simulink model "[Simulink]LA Mendoza20211984"  (R2023a)
settings: Solver=VariableStepAuto  StartTime=0.0  StopTime=10.0  RelTol=1e-3
settings Model: Creator=Marco  LastModifiedBy=Marco

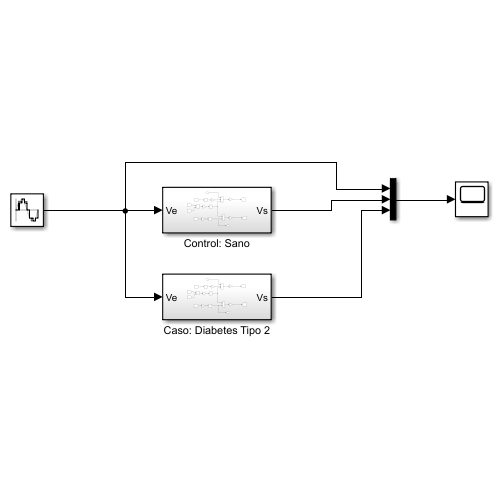
[thumbnail: Simulink's stored preview of the top-level diagram]
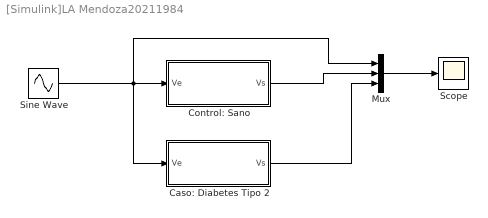
== system [Simulink]LA Mendoza20211984 ==
  Caso: Diabetes Tipo 2 : Subsystem
  Control: Sano : Subsystem
  Mux : Mux  Inputs=3
  Scope : Scope
  Sine Wave : Sin  Frequency=1.5708  SampleTime=0.001
  wires:
  Sine Wave/1 -> Caso: Diabetes Tipo 2/1(Ve), Mux/1, Control: Sano/1(Ve)
  Control: Sano/1(Vs) -> Mux/2
  Mux/1 -> Scope/1
  Caso: Diabetes Tipo 2/1(Vs) -> Mux/3

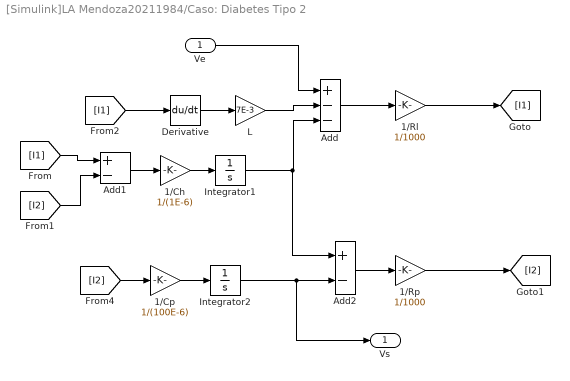
== system [Simulink]LA Mendoza20211984/Caso: Diabetes Tipo 2 ==
  Ve : Inport
  1/Ch : Gain  Gain=1/(1E-6)
  1/Cp : Gain  Gain=1/(100E-6)
  1/Rl : Gain  Gain=1/1000
  1/Rp : Gain  Gain=1/1000
  Add : Sum  Inputs=+--
  Add1 : Sum  Inputs=+-
  Add2 : Sum  Inputs=+-
  Derivative : Derivative
  Integrator1 : Integrator
  Integrator2 : Integrator
  L : Gain  Gain=7E-3
  Vs : Outport
  wires:
  Ve/1 -> Add/1
  Add1/1 -> 1/Ch/1
  [I1] -> Add1/1
  [I2] -> Add1/2
  [I1] -> Derivative/1
  Add/1 -> 1/Rl/1
  1/Rl/1 -> [I1]
  1/Ch/1 -> Integrator1/1
  Integrator1/1 -> Add2/1, Add/3
  Derivative/1 -> L/1
  L/1 -> Add/2
  [I2] -> 1/Cp/1
  1/Cp/1 -> Integrator2/1
  Integrator2/1 -> Vs/1, Add2/2
  Add2/1 -> 1/Rp/1
  1/Rp/1 -> [I2]

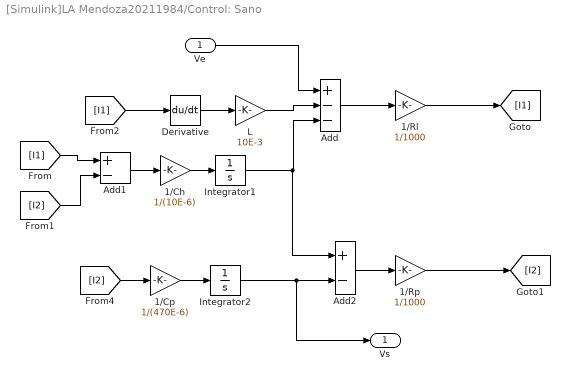
== system [Simulink]LA Mendoza20211984/Control: Sano ==
  Ve : Inport
  1/Ch : Gain  Gain=1/(10E-6)
  1/Cp : Gain  Gain=1/(470E-6)
  1/Rl : Gain  Gain=1/1000
  1/Rp : Gain  Gain=1/1000
  Add : Sum  Inputs=+--
  Add1 : Sum  Inputs=+-
  Add2 : Sum  Inputs=+-
  Derivative : Derivative
  Integrator1 : Integrator
  Integrator2 : Integrator
  L : Gain  Gain=10E-3
  Vs : Outport
  wires:
  Ve/1 -> Add/1
  Add1/1 -> 1/Ch/1
  [I1] -> Add1/1
  [I2] -> Add1/2
  [I1] -> Derivative/1
  Add/1 -> 1/Rl/1
  1/Rl/1 -> [I1]
  1/Ch/1 -> Integrator1/1
  Integrator1/1 -> Add2/1, Add/3
  Derivative/1 -> L/1
  L/1 -> Add/2
  [I2] -> 1/Cp/1
  1/Cp/1 -> Integrator2/1
  Integrator2/1 -> Vs/1, Add2/2
  Add2/1 -> 1/Rp/1
  1/Rp/1 -> [I2]
